simulink model "Observator_Kalman"  (R2020a)
settings: Solver=ode45  StartTime=0.0  StopTime=5  FixedStep=1e-3  MaxStep=1e-3  RelTol=1e-6
values from neighbouring files (symbols this model uses):
  A = [0 0 0 ; 1 0 0 ; 0 0 0]    [Initialization_Kalman.m]    (also in Kalman_Matlab.m)
  alphapoint0 = 20    [Initialization_Kalman.m]
  b = 100    [Initialization_Kalman.m]    (also in Kalman_Matlab.m = P*C')
  B = zeros(3,2)    [Initialization_Kalman.m]
  C = [1 0 1; 0 1 0]    [Initialization_Kalman.m]    (also in Kalman_Matlab.m)
  D = [0 0;0 0]    [Initialization_Kalman.m]
  F = Te*A+In    [Initialization_Kalman.m]    (also in Kalman_Matlab.m = 1/fe*A+In)
  Q = eye(3)    [Initialization_Kalman.m]    (also in Kalman_Matlab.m)
  R = 50    [Initialisation_PID.m]    (also in Initialization_Kalman.m = [Sensor_noise(1)^2 0; 0 Sensor_noise(2)^2]; Kalman_Matlab.m = [Sensor_noise(1)^2 0; 0 Sensor_noise(2)^2])
  Te = 1e-2    (= 0.01)    [Initialization_Kalman.m]
libraries: simulink x2
settings Model: Creator=Alexis  LastModifiedBy=Welcome
settings SolverCC: MaxConsecutiveMinStep=10  ShapePreserveControl=EnableAll  ZeroCrossControl=EnableAll  ZeroCrossAlgorithm=Adaptive
settings DataIOCC: ReturnWorkspaceOutputs=off
settings DebuggingCC: ArithmeticOperatorsInVariantConditions=warning
settings SFSimCC: SimUseLocalCustomCode=off  CustomCodeUndefinedFunction=UseInterfaceOnly
settings RTWCC: RTWUseLocalCustomCode=off
settings CodeAppCC: StateflowObjectComments=on

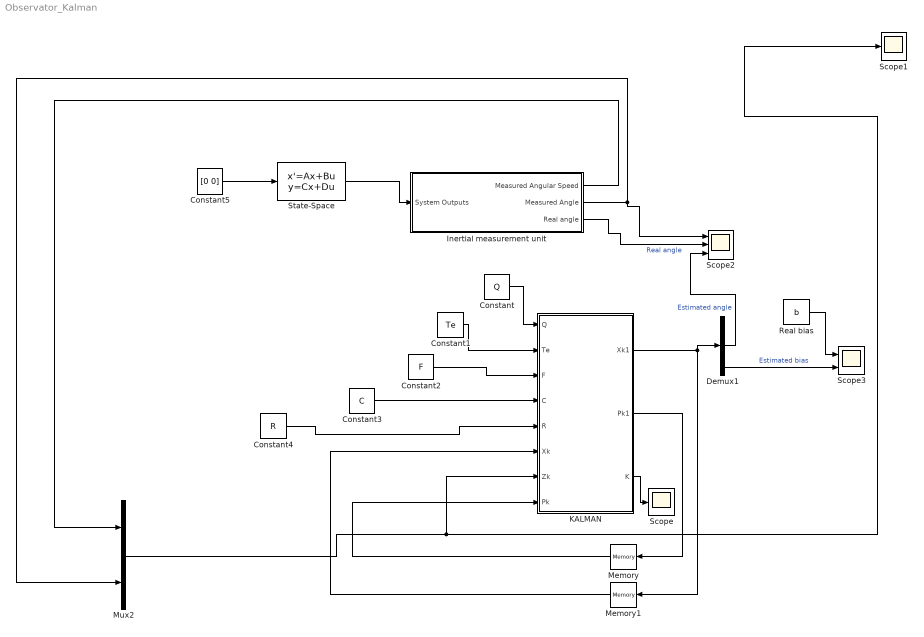
== system Observator_Kalman ==
  Constant : Constant  Value=Q
  Constant1 : Constant  Value=Te
  Constant2 : Constant  Value=F
  Constant3 : Constant  Value=C
  Constant4 : Constant  Value=R
  Constant5 : Constant  Value=[0 0]  SampleTime=Te
  Demux1 : Demux  Outputs=3
  Inertial measurement unit : Subsystem
  KALMAN : MATLAB Function  TreatAsAtomicUnit=on  SystemSampleTime=Te
  Memory : Memory  InitialCondition=eye(3)  InheritSampleTime=on
  Memory1 : Memory  InitialCondition=zeros(3,1)  InheritSampleTime=on
  Mux2 : Mux  Inputs=2
  Real bias : Constant  Value=b  SampleTime=Te
  Scope : Scope
  Scope1 : Scope
  Scope2 : Scope  NumInputPorts=3
  Scope3 : Scope  NumInputPorts=2
  State-Space : StateSpace  A=A  B=B  C=C  D=D  InitialCondition=[alphapoint0 0 b]
  wires:
  Memory/1 -> KALMAN/8(Pk)
  KALMAN/2(Pk1) -> Memory/1
  Memory1/1 -> KALMAN/6(Xk)
  KALMAN/3(K) -> Scope/1
  Constant/1 -> KALMAN/1(Q)
  Constant1/1 -> KALMAN/2(Te)
  Constant2/1 -> KALMAN/3(F)
  Constant3/1 -> KALMAN/4(C)
  Constant4/1 -> KALMAN/5(R)
  Constant5/1 -> State-Space/1
  KALMAN/1(Xk1) -> Demux1/1, Memory1/1
  Demux1/3 -> Scope3/2  "Estimated bias"
  Demux1/2 -> Scope2/3  "Estimated angle"
  Real bias/1 -> Scope3/1
  Mux2/1 -> Scope1/1, KALMAN/7(Zk)
  State-Space/1 -> Inertial measurement unit/1(System Outputs)
  Inertial measurement unit/2(Measured Angle) -> Scope2/1, Mux2/2
  Inertial measurement unit/1(Measured Angular Speed) -> Mux2/1
  Inertial measurement unit/3(Real angle) -> Scope2/2  "Real angle"

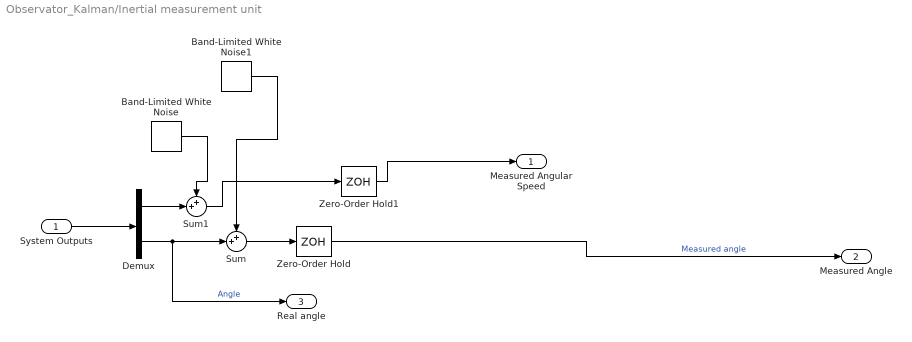
== system Observator_Kalman/Inertial measurement unit ==
  System Outputs : Inport
  Band-Limited White Noise : simulink/Sources/Band-Limited White Noise  Cov=[1E-9]  Ts=Te/10  seed=[23341]
  Band-Limited White Noise1 : simulink/Sources/Band-Limited White Noise  Cov=[1E-2]  Ts=Te/10  seed=[23341]
  Demux : Demux  Outputs=2
  Sum : Sum  Inputs=++|
  Sum1 : Sum  Inputs=++|
  Zero-Order Hold : ZeroOrderHold  SampleTime=Te
  Zero-Order Hold1 : ZeroOrderHold  SampleTime=Te
  Measured Angular Speed : Outport
  Measured Angle : Outport  Port=2
  Real angle : Outport  Port=3
  wires:
  System Outputs/1 -> Demux/1
  Demux/2 -> Real angle/1, Sum/2  "Angle"
  Sum/1 -> Zero-Order Hold/1
  Sum1/1 -> Zero-Order Hold1/1
  Demux/1 -> Sum1/2
  Band-Limited White Noise1/1 -> Sum/1
  Band-Limited White Noise/1 -> Sum1/1
  Zero-Order Hold1/1 -> Measured Angular Speed/1
  Zero-Order Hold/1 -> Measured Angle/1  "Measured angle"

== matlab function Observator_Kalman/KALMAN ==
  data: Q input; Te input; F input; C input; R input; Xk input; Xk1 output; Zk input; Pk input; Pk1 output; K output
function [Xk1,Pk1,K]  = Observator_Kalman(Q,Te,F,C,R,Xk,Zk,Pk)
Fe=1/Te;
%Prediction
Xp = F*Xk;
Pp = F*Pk*F'+Q ;%Predicted P

% Estimation
K = Fe*F*Pp*C'*((R+C*Pp*C')^(-1)) ;%Kalman gain
Pk1 = Pp-K*Te*C*Pp*F'; %Estimated P variance matrix
Xk1 = Xp + K*Te*(Zk-C*Xk);%Estimated X
